simulink model "velo_id_verify_sl"  (Simulink 8.7)
settings: Solver=ode4  StartTime=0.0  StopTime=20.0  RelTol=1e-3
values from neighbouring files (symbols this model uses):
  K = 1.57    [velo_id_verify.m]
  T = 0.76    [velo_id_verify.m]
  u_offset = 1.03    [velo_id_verify.m]
undefined symbols (not defined in the file or in its folder): p_const, r_const, ts
libraries: arduino_io_lib x4
settings Model: Creator=hirata  LastModifiedBy=masa-ito
settings DataIOCC: SignalLoggingSaveFormat=ModelDataLogs
settings OptimizationCC: ExpressionDepthLimit=2147483647
settings DebuggingCC: SolverPrmCheckMsg=warning  FcnCallInpInsideContextMsg=EnableAllAsWarning  StateNameClashWarn=warning

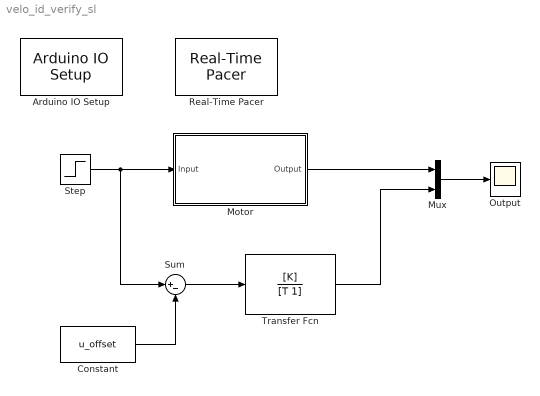
== system velo_id_verify_sl ==
  Arduino IO Setup : arduino_io_lib/Arduino IO Setup  Priority=3  arduinoVar=Temporary arduino variable: Arduino1  workspaceVarName=a  comPort=/dev/ttyS101
  Constant : Constant  Value=u_offset
  Motor : Subsystem
  Mux : Mux  Inputs=2
  Output : Scope
  Real-Time Pacer : arduino_io_lib/Real-Time Pacer  simTimePerRealTime=1
  Step : Step  Time=10  Before=r_const  After=r_const+p_const  SampleTime=ts
  Sum : Sum  Inputs=|+-
  Transfer Fcn : TransferFcn  Numerator=[K]  Denominator=[T 1]
  wires:
  Step/1 -> Motor/1(Input), Sum/1
  Sum/1 -> Transfer Fcn/1
  Constant/1 -> Sum/2
  Motor/1(Output) -> Mux/1
  Mux/1 -> Output/1
  Transfer Fcn/1 -> Mux/2

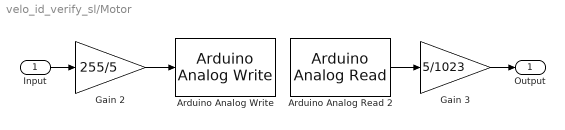
== system velo_id_verify_sl/Motor ==
  Input : Inport
  Arduino Analog Read 2 : arduino_io_lib/Arduino Analog Read  arduinoVar=Temporary arduino variable: Arduino1  arduinoPin=0  T=ts
  Arduino Analog Write : arduino_io_lib/Arduino Analog Write  arduinoVar=Temporary arduino variable: Arduino1  arduinoPin=3  T=ts
  Gain 2 : Gain  Gain=255/5
  Gain 3 : Gain  Gain=5/1023
  Output : Outport
  wires:
  Arduino Analog Read 2/1 -> Gain 3/1
  Gain 2/1 -> Arduino Analog Write/1
  Input/1 -> Gain 2/1
  Gain 3/1 -> Output/1
